simulink model "Add"  (R2015b)
settings: Solver=VariableStepAuto  StartTime=0.0  StopTime=10.0  RelTol=1e-3
settings Model: Creator=Toto  LastModifiedBy=Toto

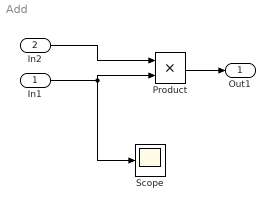
== system Add ==
  In1 : Inport
  In2 : Inport  Port=2
  Product : Product
  Scope : Scope
  Out1 : Outport
  wires:
  In2/1 -> Product/1
  In1/1 -> Scope/1, Product/2
  Product/1 -> Out1/1
